simulink model "ErskineMultiDroneFormation"  (R2020b)
settings: Solver=FixedStepAuto  StartTime=0.0  StopTime=Tsim  FixedStep=sim_dt  RelTol=1e-3
values from neighbouring files (symbols this model uses):
  controller_rate = 50    [MultiQuadInit.m]
  drone_params = setDefaultDroneParams(nDrones)    [MultiQuadInit.m]
  dt_p = 0.2    [MultiQuadInit.m]    (also in setSimConditions.m)
  edges = [1,2 ... (first row only)    [MultiQuadInit.m]    (also in setSimConditions.m)
  g = 9.81    [MultiQuadInit.m]
  N_p = 5    [MultiQuadInit.m]    (also in setSimConditions.m)
  nDrones = 3    [MultiQuadInit.m]
  omega0 = zeros(3,nDrones)    [MultiQuadInit.m]    (also in setSimConditions.m)
  p0 = scale*(rand(3,nDrones) - [0.5;0.5;0])    [MultiQuadInit.m]    (also in setSimConditions.m = scale*(rand(3,nDrones) - [1/2;1/2;0]))
  q0 = zeros(4,nDrones); q0(1,:) = ones(1,nDrones)    [MultiQuadInit.m]    (also in setSimConditions.m)
  sim_dt = 0.005    [MultiQuadInit.m]
  v0 = zeros(3, nDrones)    [MultiQuadInit.m]    (also in setSimConditions.m)
undefined symbols (not defined in the file or in its folder): camera_noise
libraries: vrlib x13
(part 4 of 4)

== matlab function ErskineMultiDroneFormation/  Quadrotor13/Quadrotor/ESC ==
  data: Omega_prop_d input; prop_acceleration output; Omega_prop input; DroneID parameter; drone_params parameter
function prop_acceleration  =  ESC_ctrl(Omega_prop_d, Omega_prop, DroneID, drone_params)

prop_acceleration = (Omega_prop_d - Omega_prop)*drone_params(DroneID).motors.gain;

== matlab function ErskineMultiDroneFormation/  Quadrotor13/Quadrotor/Translation/MATLAB Function ==
  data: f input; a output; R input; g parameter; drone_params parameter; DroneID parameter
function a = fcn(f, R, g, drone_params, DroneID)
m = drone_params(DroneID).mechanical.m;
a = R*[0;0;f]/m - [0;0;g];

== matlab function ErskineMultiDroneFormation/  Quadrotor2/Controller/Controller ==
  data: u input; p input size=3; v input size=3; q input size=4; omega input size=3; thrust output size=1; moments output size=3; control_type_param parameter; drone_params parameter; DroneID parameter; g parameter
function [thrust, moments] = controller(u, p, v, q, omega, control_type_param, drone_params, DroneID, g)

  thrust = 1; % set output dim
  moments = [0;0;0]; % set output dim
  
  coder.extrinsic('droneControl'); % link simulink to matlab function
  
  % do control
  [thrust, moments] = droneControl(u, p, v, q, omega, ...
    control_type_param, drone_params, DroneID, g);

end

== matlab function ErskineMultiDroneFormation/  Quadrotor13/Quadrotor/Translation/MATLAB Function1 ==
  data: q input; R output
function R = quat2rotm(q)
  R = eye(3);
  coder.extrinsic('quat2rotm.m');
  R = quat2rotm(q);
end

== matlab function ErskineMultiDroneFormation/  Quadrotor13/Quadrotor/calculate_wrench ==
  data: Omega_props input; thrust output; moments output; drone_params parameter; DroneID parameter
function [thrust, moments] =  invAllocation(Omega_props, drone_params, DroneID)

wrench = drone_params(DroneID).control.allocation_matrix*Omega_props.^2;

thrust = wrench(1);
moments = wrench(2:4);

== matlab function ErskineMultiDroneFormation/  Quadrotor13/add_noise ==
  settings: updateMethod=DISCRETE
  data: omega input; omega_n output size=3; q input; v input; p input; q_n output size=4; v_n output size=3; p_n output size=3; drone_params parameter; DroneID parameter
function [omega_n, q_n, v_n, p_n]= add_noise(omega,q,v,p, drone_params, DroneID)

omega_n = omega + drone_params(DroneID).sensor.gyroscope_noise*(rand(3,1)-0.5);

q_n = q + drone_params(DroneID).sensor.attitude_noise*(rand(4,1)-0.5);
q_n = q_n/norm(q_n);

v_n = v + drone_params(DroneID).sensor.velocity_noise*(rand(3,1)-0.5);

p_n = p + drone_params(DroneID).sensor.position_noise*(rand(3,1)-0.5);

end

== matlab function ErskineMultiDroneFormation/  Quadrotor2/Controller/desired_prop_speed ==
  data: thrust input; Omega_props output; moment input; drone_params parameter; DroneID parameter
function Omega_props  =  Allocation(thrust, moment, drone_params, DroneID)

%  Omega_props = sqrt(inv(alloc_mat) * [thrust;moment]);
 Omega_props = real(sqrt(complex(inv(drone_params(DroneID).control.allocation_matrix) * [thrust;moment])));

== matlab function ErskineMultiDroneFormation/  Quadrotor2/Quadrotor/Attitude/MATLAB Function ==
  data: q input size=4; omega input size=3; qd output size=4
function qd  = quaternion_derivative(q, omega)


qd =  0.5 * multiplyQuaternions([0;omega],q);

end


function q = multiplyQuaternions(qA,qB)
q0 = qA(1);
q1 = qA(2);
q2 = qA(3);
q3 = qA(4);
Q = [q0, -q1, -q2, -q3;
     q1,  q0, -q3,  q2;
     q2,  q3,  q0, -q1;
     q3, -q2,  q1,  q0];
q = Q * qB;
end

== matlab function ErskineMultiDroneFormation/  Quadrotor2/Quadrotor/Attitude/MATLAB Function1 ==
  data: m input; a output; omega input; drone_params parameter; DroneID parameter
function a = moments2angularacceleration(m, omega, drone_params, DroneID)

I = drone_params(DroneID).mechanical.I;
a = inv(I)*m  - inv(I) * cross(omega,I*omega);

== matlab function ErskineMultiDroneFormation/  Quadrotor2/Quadrotor/ESC ==
  data: Omega_prop_d input; prop_acceleration output; Omega_prop input; DroneID parameter; drone_params parameter
function prop_acceleration  =  ESC_ctrl(Omega_prop_d, Omega_prop, DroneID, drone_params)

prop_acceleration = (Omega_prop_d - Omega_prop)*drone_params(DroneID).motors.gain;

== matlab function ErskineMultiDroneFormation/  Quadrotor2/Quadrotor/Translation/MATLAB Function ==
  data: f input; a output; R input; g parameter; drone_params parameter; DroneID parameter
function a = fcn(f, R, g, drone_params, DroneID)
m = drone_params(DroneID).mechanical.m;
a = R*[0;0;f]/m - [0;0;g];

== matlab function ErskineMultiDroneFormation/Formation Controller/Camera ==
  settings: updateMethod=DISCRETE
  data: States input Bus: FormationStateBus; t input; bearings output; edges parameter; noisy_bearings output; depth output; noisy_depth output; camera_noise parameter; rng_seed parameter
function [bearings, noisy_bearings,depth, noisy_depth] = Cameras(States,t, edges, camera_noise, rng_seed)
%% Cameras(States, nDrones, edges)
% [bearings, noisy_bearings,depth, noisy_depth] = Cameras(States, nDrones, edges)

%% Setup Data Structures
drones = struct2cell(States);
bearings = zeros(3, length(edges));
noisy_bearings = zeros(3, length(edges));
depth = zeros(1, length(edges));
noisy_depth = zeros(1, length(edges));

rng(rng_seed + 1000*t);

%% Calculate Bearings
for i = 1:length(edges)
  out = edges(i,1);
  in = edges(i,2);
  
  %  drone_i = drones{out};
  %  drone_j = drones{in};
  
  Ri = quat2rotm(drones{out}.q');
  dp = drones{in}.p - drones{out}.p;
  depth(i) = norm(dp);
  bearings(:,i) = Ri' * dp/depth(i);
  
  % add noise
  perp1 = cross(bearings(:,i),rand(3,1));
  perp1 = perp1/norm(perp1);
  perp2 = cross(bearings(:,i),perp1);
  perp2 = perp2/norm(perp2);
  n1 = camera_noise.perp*2*(rand(1)-0.5)*perp1;
  n2 = camera_noise.perp*2*(rand(1)-0.5)*perp2;
  noisy_bearings(:,i) = bearings(:,i) + n1 + n2;
  noisy_bearings(:,i) = noisy_bearings(:,i)/norm(noisy_bearings(:,i));
  
  noisy_depth(i) = depth(i) + camera_noise.long_bias + ...
    2*camera_noise.long*(rand(1) - 0.5);
end

end

== matlab function ErskineMultiDroneFormation/  Quadrotor3/Controller/desired_prop_speed ==
  data: thrust input; Omega_props output; moment input; drone_params parameter; DroneID parameter
function Omega_props  =  Allocation(thrust, moment, drone_params, DroneID)

%  Omega_props = sqrt(inv(alloc_mat) * [thrust;moment]);
 Omega_props = real(sqrt(complex(inv(drone_params(DroneID).control.allocation_matrix) * [thrust;moment])));

== matlab function ErskineMultiDroneFormation/  Quadrotor3/Quadrotor/Attitude/MATLAB Function ==
  data: q input size=4; omega input size=3; qd output size=4
function qd  = quaternion_derivative(q, omega)


qd =  0.5 * multiplyQuaternions([0;omega],q);

end


function q = multiplyQuaternions(qA,qB)
q0 = qA(1);
q1 = qA(2);
q2 = qA(3);
q3 = qA(4);
Q = [q0, -q1, -q2, -q3;
     q1,  q0, -q3,  q2;
     q2,  q3,  q0, -q1;
     q3, -q2,  q1,  q0];
q = Q * qB;
end

== matlab function ErskineMultiDroneFormation/  Quadrotor3/Quadrotor/Attitude/MATLAB Function1 ==
  data: m input; a output; omega input; drone_params parameter; DroneID parameter
function a = moments2angularacceleration(m, omega, drone_params, DroneID)

I = drone_params(DroneID).mechanical.I;
a = inv(I)*m  - inv(I) * cross(omega,I*omega);

== matlab function ErskineMultiDroneFormation/  Quadrotor3/Quadrotor/ESC ==
  data: Omega_prop_d input; prop_acceleration output; Omega_prop input; DroneID parameter; drone_params parameter
function prop_acceleration  =  ESC_ctrl(Omega_prop_d, Omega_prop, DroneID, drone_params)

prop_acceleration = (Omega_prop_d - Omega_prop)*drone_params(DroneID).motors.gain;

== matlab function ErskineMultiDroneFormation/  Quadrotor1/Controller/Controller ==
  data: u input; p input size=3; v input size=3; q input size=4; omega input size=3; thrust output size=1; moments output size=3; control_type_param parameter; drone_params parameter; DroneID parameter; g parameter
function [thrust, moments] = controller(u, p, v, q, omega, control_type_param, drone_params, DroneID, g)

  thrust = 1; % set output dim
  moments = [0;0;0]; % set output dim
  
  coder.extrinsic('droneControl'); % link simulink to matlab function
  
  % do control
  [thrust, moments] = droneControl(u, p, v, q, omega, ...
    control_type_param, drone_params, DroneID, g);

end

== matlab function ErskineMultiDroneFormation/  Quadrotor3/Quadrotor/Translation/MATLAB Function ==
  data: f input; a output; R input; g parameter; drone_params parameter; DroneID parameter
function a = fcn(f, R, g, drone_params, DroneID)
m = drone_params(DroneID).mechanical.m;
a = R*[0;0;f]/m - [0;0;g];

== matlab function ErskineMultiDroneFormation/  Quadrotor3/Quadrotor/Translation/MATLAB Function1 ==
  data: q input; R output
function R = quat2rotm(q)
  R = eye(3);
  coder.extrinsic('quat2rotm.m');
  R = quat2rotm(q);
end

== matlab function ErskineMultiDroneFormation/  Quadrotor3/Quadrotor/calculate_wrench ==
  data: Omega_props input; thrust output; moments output; drone_params parameter; DroneID parameter
function [thrust, moments] =  invAllocation(Omega_props, drone_params, DroneID)

wrench = drone_params(DroneID).control.allocation_matrix*Omega_props.^2;

thrust = wrench(1);
moments = wrench(2:4);

== matlab function ErskineMultiDroneFormation/  Quadrotor3/add_noise ==
  settings: updateMethod=DISCRETE
  data: omega input; omega_n output size=3; q input; v input; p input; q_n output size=4; v_n output size=3; p_n output size=3; drone_params parameter; DroneID parameter
function [omega_n, q_n, v_n, p_n]= add_noise(omega,q,v,p, drone_params, DroneID)

omega_n = omega + drone_params(DroneID).sensor.gyroscope_noise*(rand(3,1)-0.5);

q_n = q + drone_params(DroneID).sensor.attitude_noise*(rand(4,1)-0.5);
q_n = q_n/norm(q_n);

v_n = v + drone_params(DroneID).sensor.velocity_noise*(rand(3,1)-0.5);

p_n = p + drone_params(DroneID).sensor.position_noise*(rand(3,1)-0.5);

end

== matlab function ErskineMultiDroneFormation/Formation Controller/FormationControlFunction ==
  data: states input Bus: FormationStateBus; out output size=[4*nDrones]; B_desired input; B_forward input; B_measure input; d_measure input; init_guess input; nDrones parameter; result output; N_p parameter; dt_p parameter; edges parameter; control_type parameter
function [out, result] = FormationControlFunction(states, B_desired, B_forward, B_measure, d_measure, init_guess, nDrones, N_p, dt_p, edges, control_type)
%% ControlFunction
% the control u of a drone consists of [fz; omega]
% the output of this block is  out = [u1; u2; un]
% the result of a drone is [fz1; omega1; ...; fzn, omegan]
% the result of thisblock is [result1; ...; resultn]

% Determine if first iteration
if max(init_guess) < 0.001
  first_iter = true;
else
  first_iter = false;
end


% Function variables setup
out = zeros(nDrones*4,1);
result = init_guess;

coder.extrinsic('GradientBearingController');
coder.extrinsic('ForwardMPCFormationControl');
coder.extrinsic('CommunicatingMPCFormationControl');


%% Do Control
if control_type == 1 % Gradient Controller
  if first_iter
    disp(['Control type: Gradient'])
  end
  out = GradientBearingController(B_measure, B_desired, states, nDrones, edges);
  result = ones(nDrones*4*N_p, 1);
elseif control_type == 2 % Forward Desired MPC
  if first_iter
    for i = 1:4:length(init_guess)
      init_guess(i) = 10;
    end
    disp(['Control type: Forward MPC'])
  end
  [out, result] = ForwardMPCFormationControl(states, B_forward, B_measure, d_measure, init_guess, nDrones, N_p, dt_p, edges);
elseif control_type == 3 % Forward Desired MPC with Communication
  if first_iter
    for i = 1:4:length(init_guess)
      init_guess(i) = 10;
    end
    disp(['Control type: Forward MPC with Full Communication'])
  end
  [out, result] = CommunicatingMPCFormationControl(states, B_forward, B_measure, d_measure, init_guess, nDrones, N_p, dt_p, edges);
else
  error("Chosen Control Type is Invalid")
end


%% Processing of Results

return

== matlab function ErskineMultiDroneFormation/  Quadrotor2/Quadrotor/Translation/MATLAB Function1 ==
  data: q input; R output
function R = quat2rotm(q)
  R = eye(3);
  coder.extrinsic('quat2rotm.m');
  R = quat2rotm(q);
end

== matlab function ErskineMultiDroneFormation/  Quadrotor2/Quadrotor/calculate_wrench ==
  data: Omega_props input; thrust output; moments output; drone_params parameter; DroneID parameter
function [thrust, moments] =  invAllocation(Omega_props, drone_params, DroneID)

wrench = drone_params(DroneID).control.allocation_matrix*Omega_props.^2;

thrust = wrench(1);
moments = wrench(2:4);

== matlab function ErskineMultiDroneFormation/  Quadrotor2/add_noise ==
  settings: updateMethod=DISCRETE
  data: omega input; omega_n output size=3; q input; v input; p input; q_n output size=4; v_n output size=3; p_n output size=3; drone_params parameter; DroneID parameter
function [omega_n, q_n, v_n, p_n]= add_noise(omega,q,v,p, drone_params, DroneID)

omega_n = omega + drone_params(DroneID).sensor.gyroscope_noise*(rand(3,1)-0.5);

q_n = q + drone_params(DroneID).sensor.attitude_noise*(rand(4,1)-0.5);
q_n = q_n/norm(q_n);

v_n = v + drone_params(DroneID).sensor.velocity_noise*(rand(3,1)-0.5);

p_n = p + drone_params(DroneID).sensor.position_noise*(rand(3,1)-0.5);

end

== matlab function ErskineMultiDroneFormation/  Quadrotor4/Controller/Controller ==
  data: u input; p input size=3; v input size=3; q input size=4; omega input size=3; thrust output size=1; moments output size=3; control_type_param parameter; drone_params parameter; DroneID parameter; g parameter
function [thrust, moments] = controller(u, p, v, q, omega, control_type_param, drone_params, DroneID, g)

  thrust = 1; % set output dim
  moments = [0;0;0]; % set output dim
  
  coder.extrinsic('droneControl'); % link simulink to matlab function
  
  % do control
  [thrust, moments] = droneControl(u, p, v, q, omega, ...
    control_type_param, drone_params, DroneID, g);

end

== matlab function ErskineMultiDroneFormation/  Quadrotor4/Controller/desired_prop_speed ==
  data: thrust input; Omega_props output; moment input; drone_params parameter; DroneID parameter
function Omega_props  =  Allocation(thrust, moment, drone_params, DroneID)

%  Omega_props = sqrt(inv(alloc_mat) * [thrust;moment]);
 Omega_props = real(sqrt(complex(inv(drone_params(DroneID).control.allocation_matrix) * [thrust;moment])));

== matlab function ErskineMultiDroneFormation/  Quadrotor4/Quadrotor/Attitude/MATLAB Function ==
  data: q input size=4; omega input size=3; qd output size=4
function qd  = quaternion_derivative(q, omega)


qd =  0.5 * multiplyQuaternions([0;omega],q);

end


function q = multiplyQuaternions(qA,qB)
q0 = qA(1);
q1 = qA(2);
q2 = qA(3);
q3 = qA(4);
Q = [q0, -q1, -q2, -q3;
     q1,  q0, -q3,  q2;
     q2,  q3,  q0, -q1;
     q3, -q2,  q1,  q0];
q = Q * qB;
end

== matlab function ErskineMultiDroneFormation/  Quadrotor4/Quadrotor/Attitude/MATLAB Function1 ==
  data: m input; a output; omega input; drone_params parameter; DroneID parameter
function a = moments2angularacceleration(m, omega, drone_params, DroneID)

I = drone_params(DroneID).mechanical.I;
a = inv(I)*m  - inv(I) * cross(omega,I*omega);

== matlab function ErskineMultiDroneFormation/  Quadrotor4/Quadrotor/ESC ==
  data: Omega_prop_d input; prop_acceleration output; Omega_prop input; DroneID parameter; drone_params parameter
function prop_acceleration  =  ESC_ctrl(Omega_prop_d, Omega_prop, DroneID, drone_params)

prop_acceleration = (Omega_prop_d - Omega_prop)*drone_params(DroneID).motors.gain;

== matlab function ErskineMultiDroneFormation/  Quadrotor4/Quadrotor/Translation/MATLAB Function ==
  data: f input; a output; R input; g parameter; drone_params parameter; DroneID parameter
function a = fcn(f, R, g, drone_params, DroneID)
m = drone_params(DroneID).mechanical.m;
a = R*[0;0;f]/m - [0;0;g];

== matlab function ErskineMultiDroneFormation/  Quadrotor1/Controller/desired_prop_speed ==
  data: thrust input; Omega_props output; moment input; drone_params parameter; DroneID parameter
function Omega_props  =  Allocation(thrust, moment, drone_params, DroneID)

%  Omega_props = sqrt(inv(alloc_mat) * [thrust;moment]);
 Omega_props = real(sqrt(complex(inv(drone_params(DroneID).control.allocation_matrix) * [thrust;moment])));

== matlab function ErskineMultiDroneFormation/  Quadrotor4/Quadrotor/Translation/MATLAB Function1 ==
  data: q input; R output
function R = quat2rotm(q)
  R = eye(3);
  coder.extrinsic('quat2rotm.m');
  R = quat2rotm(q);
end

== matlab function ErskineMultiDroneFormation/  Quadrotor4/Quadrotor/calculate_wrench ==
  data: Omega_props input; thrust output; moments output; drone_params parameter; DroneID parameter
function [thrust, moments] =  invAllocation(Omega_props, drone_params, DroneID)

wrench = drone_params(DroneID).control.allocation_matrix*Omega_props.^2;

thrust = wrench(1);
moments = wrench(2:4);

== matlab function ErskineMultiDroneFormation/  Quadrotor4/add_noise ==
  settings: updateMethod=DISCRETE
  data: omega input; omega_n output size=3; q input; v input; p input; q_n output size=4; v_n output size=3; p_n output size=3; drone_params parameter; DroneID parameter
function [omega_n, q_n, v_n, p_n]= add_noise(omega,q,v,p, drone_params, DroneID)

omega_n = omega + drone_params(DroneID).sensor.gyroscope_noise*(rand(3,1)-0.5);

q_n = q + drone_params(DroneID).sensor.attitude_noise*(rand(4,1)-0.5);
q_n = q_n/norm(q_n);

v_n = v + drone_params(DroneID).sensor.velocity_noise*(rand(3,1)-0.5);

p_n = p + drone_params(DroneID).sensor.position_noise*(rand(3,1)-0.5);

end

== matlab function ErskineMultiDroneFormation/  Quadrotor5/Controller/Controller ==
  data: u input; p input size=3; v input size=3; q input size=4; omega input size=3; thrust output size=1; moments output size=3; control_type_param parameter; drone_params parameter; DroneID parameter; g parameter
function [thrust, moments] = controller(u, p, v, q, omega, control_type_param, drone_params, DroneID, g)

  thrust = 1; % set output dim
  moments = [0;0;0]; % set output dim
  
  coder.extrinsic('droneControl'); % link simulink to matlab function
  
  % do control
  [thrust, moments] = droneControl(u, p, v, q, omega, ...
    control_type_param, drone_params, DroneID, g);

end

== matlab function ErskineMultiDroneFormation/  Quadrotor5/Controller/desired_prop_speed ==
  data: thrust input; Omega_props output; moment input; drone_params parameter; DroneID parameter
function Omega_props  =  Allocation(thrust, moment, drone_params, DroneID)

%  Omega_props = sqrt(inv(alloc_mat) * [thrust;moment]);
 Omega_props = real(sqrt(complex(inv(drone_params(DroneID).control.allocation_matrix) * [thrust;moment])));

== matlab function ErskineMultiDroneFormation/  Quadrotor5/Quadrotor/Attitude/MATLAB Function ==
  data: q input size=4; omega input size=3; qd output size=4
function qd  = quaternion_derivative(q, omega)


qd =  0.5 * multiplyQuaternions([0;omega],q);

end


function q = multiplyQuaternions(qA,qB)
q0 = qA(1);
q1 = qA(2);
q2 = qA(3);
q3 = qA(4);
Q = [q0, -q1, -q2, -q3;
     q1,  q0, -q3,  q2;
     q2,  q3,  q0, -q1;
     q3, -q2,  q1,  q0];
q = Q * qB;
end

== matlab function ErskineMultiDroneFormation/  Quadrotor5/Quadrotor/Attitude/MATLAB Function1 ==
  data: m input; a output; omega input; drone_params parameter; DroneID parameter
function a = moments2angularacceleration(m, omega, drone_params, DroneID)

I = drone_params(DroneID).mechanical.I;
a = inv(I)*m  - inv(I) * cross(omega,I*omega);

== matlab function ErskineMultiDroneFormation/  Quadrotor5/Quadrotor/ESC ==
  data: Omega_prop_d input; prop_acceleration output; Omega_prop input; DroneID parameter; drone_params parameter
function prop_acceleration  =  ESC_ctrl(Omega_prop_d, Omega_prop, DroneID, drone_params)

prop_acceleration = (Omega_prop_d - Omega_prop)*drone_params(DroneID).motors.gain;

== matlab function ErskineMultiDroneFormation/  Quadrotor5/Quadrotor/Translation/MATLAB Function ==
  data: f input; a output; R input; g parameter; drone_params parameter; DroneID parameter
function a = fcn(f, R, g, drone_params, DroneID)
m = drone_params(DroneID).mechanical.m;
a = R*[0;0;f]/m - [0;0;g];

== matlab function ErskineMultiDroneFormation/  Quadrotor1/Quadrotor/Attitude/MATLAB Function ==
  data: q input size=4; omega input size=3; qd output size=4
function qd  = quaternion_derivative(q, omega)


qd =  0.5 * multiplyQuaternions([0;omega],q);

end


function q = multiplyQuaternions(qA,qB)
q0 = qA(1);
q1 = qA(2);
q2 = qA(3);
q3 = qA(4);
Q = [q0, -q1, -q2, -q3;
     q1,  q0, -q3,  q2;
     q2,  q3,  q0, -q1;
     q3, -q2,  q1,  q0];
q = Q * qB;
end

== matlab function ErskineMultiDroneFormation/  Quadrotor5/Quadrotor/Translation/MATLAB Function1 ==
  data: q input; R output
function R = quat2rotm(q)
  R = eye(3);
  coder.extrinsic('quat2rotm.m');
  R = quat2rotm(q);
end

== matlab function ErskineMultiDroneFormation/  Quadrotor5/Quadrotor/calculate_wrench ==
  data: Omega_props input; thrust output; moments output; drone_params parameter; DroneID parameter
function [thrust, moments] =  invAllocation(Omega_props, drone_params, DroneID)

wrench = drone_params(DroneID).control.allocation_matrix*Omega_props.^2;

thrust = wrench(1);
moments = wrench(2:4);

== matlab function ErskineMultiDroneFormation/  Quadrotor5/add_noise ==
  settings: updateMethod=DISCRETE
  data: omega input; omega_n output size=3; q input; v input; p input; q_n output size=4; v_n output size=3; p_n output size=3; drone_params parameter; DroneID parameter
function [omega_n, q_n, v_n, p_n]= add_noise(omega,q,v,p, drone_params, DroneID)

omega_n = omega + drone_params(DroneID).sensor.gyroscope_noise*(rand(3,1)-0.5);

q_n = q + drone_params(DroneID).sensor.attitude_noise*(rand(4,1)-0.5);
q_n = q_n/norm(q_n);

v_n = v + drone_params(DroneID).sensor.velocity_noise*(rand(3,1)-0.5);

p_n = p + drone_params(DroneID).sensor.position_noise*(rand(3,1)-0.5);

end

== matlab function ErskineMultiDroneFormation/  Quadrotor6/Controller/Controller ==
  data: u input; p input size=3; v input size=3; q input size=4; omega input size=3; thrust output size=1; moments output size=3; control_type_param parameter; drone_params parameter; DroneID parameter; g parameter
function [thrust, moments] = controller(u, p, v, q, omega, control_type_param, drone_params, DroneID, g)

  thrust = 1; % set output dim
  moments = [0;0;0]; % set output dim
  
  coder.extrinsic('droneControl'); % link simulink to matlab function
  
  % do control
  [thrust, moments] = droneControl(u, p, v, q, omega, ...
    control_type_param, drone_params, DroneID, g);

end

== matlab function ErskineMultiDroneFormation/  Quadrotor6/Controller/desired_prop_speed ==
  data: thrust input; Omega_props output; moment input; drone_params parameter; DroneID parameter
function Omega_props  =  Allocation(thrust, moment, drone_params, DroneID)

%  Omega_props = sqrt(inv(alloc_mat) * [thrust;moment]);
 Omega_props = real(sqrt(complex(inv(drone_params(DroneID).control.allocation_matrix) * [thrust;moment])));

== matlab function ErskineMultiDroneFormation/  Quadrotor6/Quadrotor/Attitude/MATLAB Function ==
  data: q input size=4; omega input size=3; qd output size=4
function qd  = quaternion_derivative(q, omega)


qd =  0.5 * multiplyQuaternions([0;omega],q);

end


function q = multiplyQuaternions(qA,qB)
q0 = qA(1);
q1 = qA(2);
q2 = qA(3);
q3 = qA(4);
Q = [q0, -q1, -q2, -q3;
     q1,  q0, -q3,  q2;
     q2,  q3,  q0, -q1;
     q3, -q2,  q1,  q0];
q = Q * qB;
end

== matlab function ErskineMultiDroneFormation/  Quadrotor6/Quadrotor/Attitude/MATLAB Function1 ==
  data: m input; a output; omega input; drone_params parameter; DroneID parameter
function a = moments2angularacceleration(m, omega, drone_params, DroneID)

I = drone_params(DroneID).mechanical.I;
a = inv(I)*m  - inv(I) * cross(omega,I*omega);

== matlab function ErskineMultiDroneFormation/  Quadrotor6/Quadrotor/ESC ==
  data: Omega_prop_d input; prop_acceleration output; Omega_prop input; DroneID parameter; drone_params parameter
function prop_acceleration  =  ESC_ctrl(Omega_prop_d, Omega_prop, DroneID, drone_params)

prop_acceleration = (Omega_prop_d - Omega_prop)*drone_params(DroneID).motors.gain;

== matlab function ErskineMultiDroneFormation/  Quadrotor1/Quadrotor/Attitude/MATLAB Function1 ==
  data: m input; a output; omega input; drone_params parameter; DroneID parameter
function a = moments2angularacceleration(m, omega, drone_params, DroneID)

I = drone_params(DroneID).mechanical.I;
a = inv(I)*m  - inv(I) * cross(omega,I*omega);

== matlab function ErskineMultiDroneFormation/  Quadrotor6/Quadrotor/Translation/MATLAB Function ==
  data: f input; a output; R input; g parameter; drone_params parameter; DroneID parameter
function a = fcn(f, R, g, drone_params, DroneID)
m = drone_params(DroneID).mechanical.m;
a = R*[0;0;f]/m - [0;0;g];

== matlab function ErskineMultiDroneFormation/  Quadrotor6/Quadrotor/Translation/MATLAB Function1 ==
  data: q input; R output
function R = quat2rotm(q)
  R = eye(3);
  coder.extrinsic('quat2rotm.m');
  R = quat2rotm(q);
end

== matlab function ErskineMultiDroneFormation/  Quadrotor6/Quadrotor/calculate_wrench ==
  data: Omega_props input; thrust output; moments output; drone_params parameter; DroneID parameter
function [thrust, moments] =  invAllocation(Omega_props, drone_params, DroneID)

wrench = drone_params(DroneID).control.allocation_matrix*Omega_props.^2;

thrust = wrench(1);
moments = wrench(2:4);

== matlab function ErskineMultiDroneFormation/  Quadrotor6/add_noise ==
  settings: updateMethod=DISCRETE
  data: omega input; omega_n output size=3; q input; v input; p input; q_n output size=4; v_n output size=3; p_n output size=3; drone_params parameter; DroneID parameter
function [omega_n, q_n, v_n, p_n]= add_noise(omega,q,v,p, drone_params, DroneID)

omega_n = omega + drone_params(DroneID).sensor.gyroscope_noise*(rand(3,1)-0.5);

q_n = q + drone_params(DroneID).sensor.attitude_noise*(rand(4,1)-0.5);
q_n = q_n/norm(q_n);

v_n = v + drone_params(DroneID).sensor.velocity_noise*(rand(3,1)-0.5);

p_n = p + drone_params(DroneID).sensor.position_noise*(rand(3,1)-0.5);

end

== matlab function ErskineMultiDroneFormation/Formation Controller1/Camera ==
  settings: updateMethod=DISCRETE
  data: States input Bus: FormationStateBus; t input; bearings output; edges parameter; noisy_bearings output; depth output; noisy_depth output; camera_noise parameter; rng_seed parameter
function [bearings, noisy_bearings,depth, noisy_depth] = Cameras(States,t, edges, camera_noise, rng_seed)
%% Cameras(States, nDrones, edges)
% [bearings, noisy_bearings,depth, noisy_depth] = Cameras(States, nDrones, edges)

%% Setup Data Structures
drones = struct2cell(States);
bearings = zeros(3, length(edges));
noisy_bearings = zeros(3, length(edges));
depth = zeros(1, length(edges));
noisy_depth = zeros(1, length(edges));

rng(rng_seed + 1000*t);

%% Calculate Bearings
for i = 1:length(edges)
  out = edges(i,1);
  in = edges(i,2);
  
  %  drone_i = drones{out};
  %  drone_j = drones{in};
  
  Ri = quat2rotm(drones{out}.q');
  dp = drones{in}.p - drones{out}.p;
  depth(i) = norm(dp);
  bearings(:,i) = Ri' * dp/depth(i);
  
  % add noise
  perp1 = cross(bearings(:,i),rand(3,1));
  perp1 = perp1/norm(perp1);
  perp2 = cross(bearings(:,i),perp1);
  perp2 = perp2/norm(perp2);
  n1 = camera_noise.perp*2*(rand(1)-0.5)*perp1;
  n2 = camera_noise.perp*2*(rand(1)-0.5)*perp2;
  noisy_bearings(:,i) = bearings(:,i) + n1 + n2;
  noisy_bearings(:,i) = noisy_bearings(:,i)/norm(noisy_bearings(:,i));
  
  noisy_depth(i) = depth(i) + camera_noise.long_bias + ...
    2*camera_noise.long*(rand(1) - 0.5);
end

end

== matlab function ErskineMultiDroneFormation/Formation Controller1/FormationControlFunction ==
  data: states input Bus: FormationStateBus; out output size=[4*nDrones]; B_desired input; B_forward input; B_measure input; d_measure input; init_guess input; nDrones parameter; result output; N_p parameter; dt_p parameter; edges parameter; control_type parameter
function [out, result] = FormationControlFunction(states, B_desired, B_forward, B_measure, d_measure, init_guess, nDrones, N_p, dt_p, edges, control_type)
%% ControlFunction
% the control u of a drone consists of [fz; omega]
% the output of this block is  out = [u1; u2; un]
% the result of a drone is [fz1; omega1; ...; fzn, omegan]
% the result of thisblock is [result1; ...; resultn]

% Determine if first iteration
if max(init_guess) < 0.001
  first_iter = true;
else
  first_iter = false;
end


% Function variables setup
out = zeros(nDrones*4,1);
result = init_guess;

coder.extrinsic('GradientBearingController');
coder.extrinsic('ForwardMPCFormationControl');
coder.extrinsic('CommunicatingMPCFormationControl');


%% Do Control
if control_type == 1 % Gradient Controller
  if first_iter
    disp(['Control type: Gradient'])
  end
  out = GradientBearingController(B_measure, B_desired, states, nDrones, edges);
  result = ones(nDrones*4*N_p, 1);
elseif control_type == 2 % Forward Desired MPC
  if first_iter
    for i = 1:4:length(init_guess)
      init_guess(i) = 10;
    end
    disp(['Control type: Forward MPC'])
  end
  [out, result] = ForwardMPCFormationControl(states, B_forward, B_measure, d_measure, init_guess, nDrones, N_p, dt_p, edges);
elseif control_type == 3 % Forward Desired MPC with Communication
  if first_iter
    for i = 1:4:length(init_guess)
      init_guess(i) = 10;
    end
    disp(['Control type: Forward MPC with Full Communication'])
  end
  [out, result] = CommunicatingMPCFormationControl(states, B_forward, B_measure, d_measure, init_guess, nDrones, N_p, dt_p, edges);
else
  error("Chosen Control Type is Invalid")
end


%% Processing of Results

return

== matlab function ErskineMultiDroneFormation/  Quadrotor7/Controller/Controller ==
  data: u input; p input size=3; v input size=3; q input size=4; omega input size=3; thrust output size=1; moments output size=3; control_type_param parameter; drone_params parameter; DroneID parameter; g parameter
function [thrust, moments] = controller(u, p, v, q, omega, control_type_param, drone_params, DroneID, g)

  thrust = 1; % set output dim
  moments = [0;0;0]; % set output dim
  
  coder.extrinsic('droneControl'); % link simulink to matlab function
  
  % do control
  [thrust, moments] = droneControl(u, p, v, q, omega, ...
    control_type_param, drone_params, DroneID, g);

end

== matlab function ErskineMultiDroneFormation/  Quadrotor7/Controller/desired_prop_speed ==
  data: thrust input; Omega_props output; moment input; drone_params parameter; DroneID parameter
function Omega_props  =  Allocation(thrust, moment, drone_params, DroneID)

%  Omega_props = sqrt(inv(alloc_mat) * [thrust;moment]);
 Omega_props = real(sqrt(complex(inv(drone_params(DroneID).control.allocation_matrix) * [thrust;moment])));

== matlab function ErskineMultiDroneFormation/  Quadrotor1/Quadrotor/ESC ==
  data: Omega_prop_d input; prop_acceleration output; Omega_prop input; DroneID parameter; drone_params parameter
function prop_acceleration  =  ESC_ctrl(Omega_prop_d, Omega_prop, DroneID, drone_params)

prop_acceleration = (Omega_prop_d - Omega_prop)*drone_params(DroneID).motors.gain;

== matlab function ErskineMultiDroneFormation/  Quadrotor7/Quadrotor/Attitude/MATLAB Function ==
  data: q input size=4; omega input size=3; qd output size=4
function qd  = quaternion_derivative(q, omega)


qd =  0.5 * multiplyQuaternions([0;omega],q);

end


function q = multiplyQuaternions(qA,qB)
q0 = qA(1);
q1 = qA(2);
q2 = qA(3);
q3 = qA(4);
Q = [q0, -q1, -q2, -q3;
     q1,  q0, -q3,  q2;
     q2,  q3,  q0, -q1;
     q3, -q2,  q1,  q0];
q = Q * qB;
end

== matlab function ErskineMultiDroneFormation/  Quadrotor7/Quadrotor/Attitude/MATLAB Function1 ==
  data: m input; a output; omega input; drone_params parameter; DroneID parameter
function a = moments2angularacceleration(m, omega, drone_params, DroneID)

I = drone_params(DroneID).mechanical.I;
a = inv(I)*m  - inv(I) * cross(omega,I*omega);

== matlab function ErskineMultiDroneFormation/  Quadrotor7/Quadrotor/ESC ==
  data: Omega_prop_d input; prop_acceleration output; Omega_prop input; DroneID parameter; drone_params parameter
function prop_acceleration  =  ESC_ctrl(Omega_prop_d, Omega_prop, DroneID, drone_params)

prop_acceleration = (Omega_prop_d - Omega_prop)*drone_params(DroneID).motors.gain;

== matlab function ErskineMultiDroneFormation/  Quadrotor7/Quadrotor/Translation/MATLAB Function ==
  data: f input; a output; R input; g parameter; drone_params parameter; DroneID parameter
function a = fcn(f, R, g, drone_params, DroneID)
m = drone_params(DroneID).mechanical.m;
a = R*[0;0;f]/m - [0;0;g];

== matlab function ErskineMultiDroneFormation/  Quadrotor7/Quadrotor/Translation/MATLAB Function1 ==
  data: q input; R output
function R = quat2rotm(q)
  R = eye(3);
  coder.extrinsic('quat2rotm.m');
  R = quat2rotm(q);
end

== matlab function ErskineMultiDroneFormation/  Quadrotor7/Quadrotor/calculate_wrench ==
  data: Omega_props input; thrust output; moments output; drone_params parameter; DroneID parameter
function [thrust, moments] =  invAllocation(Omega_props, drone_params, DroneID)

wrench = drone_params(DroneID).control.allocation_matrix*Omega_props.^2;

thrust = wrench(1);
moments = wrench(2:4);

== matlab function ErskineMultiDroneFormation/  Quadrotor7/add_noise ==
  settings: updateMethod=DISCRETE
  data: omega input; omega_n output size=3; q input; v input; p input; q_n output size=4; v_n output size=3; p_n output size=3; drone_params parameter; DroneID parameter
function [omega_n, q_n, v_n, p_n]= add_noise(omega,q,v,p, drone_params, DroneID)

omega_n = omega + drone_params(DroneID).sensor.gyroscope_noise*(rand(3,1)-0.5);

q_n = q + drone_params(DroneID).sensor.attitude_noise*(rand(4,1)-0.5);
q_n = q_n/norm(q_n);

v_n = v + drone_params(DroneID).sensor.velocity_noise*(rand(3,1)-0.5);

p_n = p + drone_params(DroneID).sensor.position_noise*(rand(3,1)-0.5);

end

== matlab function ErskineMultiDroneFormation/  Quadrotor8/Controller/Controller ==
  data: u input; p input size=3; v input size=3; q input size=4; omega input size=3; thrust output size=1; moments output size=3; control_type_param parameter; drone_params parameter; DroneID parameter; g parameter
function [thrust, moments] = controller(u, p, v, q, omega, control_type_param, drone_params, DroneID, g)

  thrust = 1; % set output dim
  moments = [0;0;0]; % set output dim
  
  coder.extrinsic('droneControl'); % link simulink to matlab function
  
  % do control
  [thrust, moments] = droneControl(u, p, v, q, omega, ...
    control_type_param, drone_params, DroneID, g);

end

== matlab function ErskineMultiDroneFormation/  Quadrotor8/Controller/desired_prop_speed ==
  data: thrust input; Omega_props output; moment input; drone_params parameter; DroneID parameter
function Omega_props  =  Allocation(thrust, moment, drone_params, DroneID)

%  Omega_props = sqrt(inv(alloc_mat) * [thrust;moment]);
 Omega_props = real(sqrt(complex(inv(drone_params(DroneID).control.allocation_matrix) * [thrust;moment])));

== matlab function ErskineMultiDroneFormation/  Quadrotor1/Quadrotor/Translation/MATLAB Function ==
  data: f input; a output; R input; g parameter; drone_params parameter; DroneID parameter
function a = fcn(f, R, g, drone_params, DroneID)
m = drone_params(DroneID).mechanical.m;
a = R*[0;0;f]/m - [0;0;g];

== matlab function ErskineMultiDroneFormation/  Quadrotor8/Quadrotor/Attitude/MATLAB Function ==
  data: q input size=4; omega input size=3; qd output size=4
function qd  = quaternion_derivative(q, omega)


qd =  0.5 * multiplyQuaternions([0;omega],q);

end


function q = multiplyQuaternions(qA,qB)
q0 = qA(1);
q1 = qA(2);
q2 = qA(3);
q3 = qA(4);
Q = [q0, -q1, -q2, -q3;
     q1,  q0, -q3,  q2;
     q2,  q3,  q0, -q1;
     q3, -q2,  q1,  q0];
q = Q * qB;
end

== matlab function ErskineMultiDroneFormation/  Quadrotor8/Quadrotor/Attitude/MATLAB Function1 ==
  data: m input; a output; omega input; drone_params parameter; DroneID parameter
function a = moments2angularacceleration(m, omega, drone_params, DroneID)

I = drone_params(DroneID).mechanical.I;
a = inv(I)*m  - inv(I) * cross(omega,I*omega);

== matlab function ErskineMultiDroneFormation/  Quadrotor8/Quadrotor/ESC ==
  data: Omega_prop_d input; prop_acceleration output; Omega_prop input; DroneID parameter; drone_params parameter
function prop_acceleration  =  ESC_ctrl(Omega_prop_d, Omega_prop, DroneID, drone_params)

prop_acceleration = (Omega_prop_d - Omega_prop)*drone_params(DroneID).motors.gain;

== matlab function ErskineMultiDroneFormation/  Quadrotor8/Quadrotor/Translation/MATLAB Function ==
  data: f input; a output; R input; g parameter; drone_params parameter; DroneID parameter
function a = fcn(f, R, g, drone_params, DroneID)
m = drone_params(DroneID).mechanical.m;
a = R*[0;0;f]/m - [0;0;g];

== matlab function ErskineMultiDroneFormation/  Quadrotor8/Quadrotor/Translation/MATLAB Function1 ==
  data: q input; R output
function R = quat2rotm(q)
  R = eye(3);
  coder.extrinsic('quat2rotm.m');
  R = quat2rotm(q);
end

== matlab function ErskineMultiDroneFormation/  Quadrotor8/Quadrotor/calculate_wrench ==
  data: Omega_props input; thrust output; moments output; drone_params parameter; DroneID parameter
function [thrust, moments] =  invAllocation(Omega_props, drone_params, DroneID)

wrench = drone_params(DroneID).control.allocation_matrix*Omega_props.^2;

thrust = wrench(1);
moments = wrench(2:4);

== matlab function ErskineMultiDroneFormation/  Quadrotor8/add_noise ==
  settings: updateMethod=DISCRETE
  data: omega input; omega_n output size=3; q input; v input; p input; q_n output size=4; v_n output size=3; p_n output size=3; drone_params parameter; DroneID parameter
function [omega_n, q_n, v_n, p_n]= add_noise(omega,q,v,p, drone_params, DroneID)

omega_n = omega + drone_params(DroneID).sensor.gyroscope_noise*(rand(3,1)-0.5);

q_n = q + drone_params(DroneID).sensor.attitude_noise*(rand(4,1)-0.5);
q_n = q_n/norm(q_n);

v_n = v + drone_params(DroneID).sensor.velocity_noise*(rand(3,1)-0.5);

p_n = p + drone_params(DroneID).sensor.position_noise*(rand(3,1)-0.5);

end

== matlab function ErskineMultiDroneFormation/  Quadrotor9/Controller/Controller ==
  data: u input; p input size=3; v input size=3; q input size=4; omega input size=3; thrust output size=1; moments output size=3; control_type_param parameter; drone_params parameter; DroneID parameter; g parameter
function [thrust, moments] = controller(u, p, v, q, omega, control_type_param, drone_params, DroneID, g)

  thrust = 1; % set output dim
  moments = [0;0;0]; % set output dim
  
  coder.extrinsic('droneControl'); % link simulink to matlab function
  
  % do control
  [thrust, moments] = droneControl(u, p, v, q, omega, ...
    control_type_param, drone_params, DroneID, g);

end

== matlab function ErskineMultiDroneFormation/  Quadrotor9/Controller/desired_prop_speed ==
  data: thrust input; Omega_props output; moment input; drone_params parameter; DroneID parameter
function Omega_props  =  Allocation(thrust, moment, drone_params, DroneID)

%  Omega_props = sqrt(inv(alloc_mat) * [thrust;moment]);
 Omega_props = real(sqrt(complex(inv(drone_params(DroneID).control.allocation_matrix) * [thrust;moment])));

== matlab function ErskineMultiDroneFormation/  Quadrotor9/Quadrotor/Attitude/MATLAB Function ==
  data: q input size=4; omega input size=3; qd output size=4
function qd  = quaternion_derivative(q, omega)


qd =  0.5 * multiplyQuaternions([0;omega],q);

end


function q = multiplyQuaternions(qA,qB)
q0 = qA(1);
q1 = qA(2);
q2 = qA(3);
q3 = qA(4);
Q = [q0, -q1, -q2, -q3;
     q1,  q0, -q3,  q2;
     q2,  q3,  q0, -q1;
     q3, -q2,  q1,  q0];
q = Q * qB;
end

== matlab function ErskineMultiDroneFormation/  Quadrotor9/Quadrotor/Attitude/MATLAB Function1 ==
  data: m input; a output; omega input; drone_params parameter; DroneID parameter
function a = moments2angularacceleration(m, omega, drone_params, DroneID)

I = drone_params(DroneID).mechanical.I;
a = inv(I)*m  - inv(I) * cross(omega,I*omega);

== matlab function ErskineMultiDroneFormation/  Quadrotor1/Quadrotor/Translation/MATLAB Function1 ==
  data: q input; R output
function R = quat2rotm(q)
  R = eye(3);
  coder.extrinsic('quat2rotm.m');
  R = quat2rotm(q);
end

== matlab function ErskineMultiDroneFormation/  Quadrotor9/Quadrotor/ESC ==
  data: Omega_prop_d input; prop_acceleration output; Omega_prop input; DroneID parameter; drone_params parameter
function prop_acceleration  =  ESC_ctrl(Omega_prop_d, Omega_prop, DroneID, drone_params)

prop_acceleration = (Omega_prop_d - Omega_prop)*drone_params(DroneID).motors.gain;

== matlab function ErskineMultiDroneFormation/  Quadrotor9/Quadrotor/Translation/MATLAB Function ==
  data: f input; a output; R input; g parameter; drone_params parameter; DroneID parameter
function a = fcn(f, R, g, drone_params, DroneID)
m = drone_params(DroneID).mechanical.m;
a = R*[0;0;f]/m - [0;0;g];

== matlab function ErskineMultiDroneFormation/  Quadrotor9/Quadrotor/Translation/MATLAB Function1 ==
  data: q input; R output
function R = quat2rotm(q)
  R = eye(3);
  coder.extrinsic('quat2rotm.m');
  R = quat2rotm(q);
end

== matlab function ErskineMultiDroneFormation/  Quadrotor9/Quadrotor/calculate_wrench ==
  data: Omega_props input; thrust output; moments output; drone_params parameter; DroneID parameter
function [thrust, moments] =  invAllocation(Omega_props, drone_params, DroneID)

wrench = drone_params(DroneID).control.allocation_matrix*Omega_props.^2;

thrust = wrench(1);
moments = wrench(2:4);

== matlab function ErskineMultiDroneFormation/  Quadrotor9/add_noise ==
  settings: updateMethod=DISCRETE
  data: omega input; omega_n output size=3; q input; v input; p input; q_n output size=4; v_n output size=3; p_n output size=3; drone_params parameter; DroneID parameter
function [omega_n, q_n, v_n, p_n]= add_noise(omega,q,v,p, drone_params, DroneID)

omega_n = omega + drone_params(DroneID).sensor.gyroscope_noise*(rand(3,1)-0.5);

q_n = q + drone_params(DroneID).sensor.attitude_noise*(rand(4,1)-0.5);
q_n = q_n/norm(q_n);

v_n = v + drone_params(DroneID).sensor.velocity_noise*(rand(3,1)-0.5);

p_n = p + drone_params(DroneID).sensor.position_noise*(rand(3,1)-0.5);

end

== matlab function ErskineMultiDroneFormation/Formation Controller2/Camera ==
  settings: updateMethod=DISCRETE
  data: States input Bus: FormationStateBus; t input; bearings output; edges parameter; noisy_bearings output; depth output; noisy_depth output; camera_noise parameter; rng_seed parameter
function [bearings, noisy_bearings,depth, noisy_depth] = Cameras(States,t, edges, camera_noise, rng_seed)
%% Cameras(States, nDrones, edges)
% [bearings, noisy_bearings,depth, noisy_depth] = Cameras(States, nDrones, edges)

%% Setup Data Structures
drones = struct2cell(States);
bearings = zeros(3, length(edges));
noisy_bearings = zeros(3, length(edges));
depth = zeros(1, length(edges));
noisy_depth = zeros(1, length(edges));

rng(rng_seed + 1000*t);

%% Calculate Bearings
for i = 1:length(edges)
  out = edges(i,1);
  in = edges(i,2);
  
  %  drone_i = drones{out};
  %  drone_j = drones{in};
  
  Ri = quat2rotm(drones{out}.q');
  dp = drones{in}.p - drones{out}.p;
  depth(i) = norm(dp);
  bearings(:,i) = Ri' * dp/depth(i);
  
  % add noise
  perp1 = cross(bearings(:,i),rand(3,1));
  perp1 = perp1/norm(perp1);
  perp2 = cross(bearings(:,i),perp1);
  perp2 = perp2/norm(perp2);
  n1 = camera_noise.perp*2*(rand(1)-0.5)*perp1;
  n2 = camera_noise.perp*2*(rand(1)-0.5)*perp2;
  noisy_bearings(:,i) = bearings(:,i) + n1 + n2;
  noisy_bearings(:,i) = noisy_bearings(:,i)/norm(noisy_bearings(:,i));
  
  noisy_depth(i) = depth(i) + camera_noise.long_bias + ...
    2*camera_noise.long*(rand(1) - 0.5);
end

end

== matlab function ErskineMultiDroneFormation/  Quadrotor1/Quadrotor/calculate_wrench ==
  data: Omega_props input; thrust output; moments output; drone_params parameter; DroneID parameter
function [thrust, moments] =  invAllocation(Omega_props, drone_params, DroneID)

wrench = drone_params(DroneID).control.allocation_matrix*Omega_props.^2;

thrust = wrench(1);
moments = wrench(2:4);

== matlab function ErskineMultiDroneFormation/Formation Controller2/FormationControlFunction ==
  data: states input Bus: FormationStateBus; out output size=[4*nDrones]; B_desired input; B_forward input; B_measure input; d_measure input; init_guess input; nDrones parameter; result output; N_p parameter; dt_p parameter; edges parameter; control_type parameter
function [out, result] = FormationControlFunction(states, B_desired, B_forward, B_measure, d_measure, init_guess, nDrones, N_p, dt_p, edges, control_type)
%% ControlFunction
% the control u of a drone consists of [fz; omega]
% the output of this block is  out = [u1; u2; un]
% the result of a drone is [fz1; omega1; ...; fzn, omegan]
% the result of thisblock is [result1; ...; resultn]

% Determine if first iteration
if max(init_guess) < 0.001
  first_iter = true;
else
  first_iter = false;
end


% Function variables setup
out = zeros(nDrones*4,1);
result = init_guess;

coder.extrinsic('GradientBearingController');
coder.extrinsic('ForwardMPCFormationControl');
coder.extrinsic('CommunicatingMPCFormationControl');


%% Do Control
if control_type == 1 % Gradient Controller
  if first_iter
    disp(['Control type: Gradient'])
  end
  out = GradientBearingController(B_measure, B_desired, states, nDrones, edges);
  result = ones(nDrones*4*N_p, 1);
elseif control_type == 2 % Forward Desired MPC
  if first_iter
    for i = 1:4:length(init_guess)
      init_guess(i) = 10;
    end
    disp(['Control type: Forward MPC'])
  end
  [out, result] = ForwardMPCFormationControl(states, B_forward, B_measure, d_measure, init_guess, nDrones, N_p, dt_p, edges);
elseif control_type == 3 % Forward Desired MPC with Communication
  if first_iter
    for i = 1:4:length(init_guess)
      init_guess(i) = 10;
    end
    disp(['Control type: Forward MPC with Full Communication'])
  end
  [out, result] = CommunicatingMPCFormationControl(states, B_forward, B_measure, d_measure, init_guess, nDrones, N_p, dt_p, edges);
else
  error("Chosen Control Type is Invalid")
end


%% Processing of Results

return

== matlab function ErskineMultiDroneFormation/  Quadrotor10/Controller/Controller ==
  data: u input; p input size=3; v input size=3; q input size=4; omega input size=3; thrust output size=1; moments output size=3; control_type_param parameter; drone_params parameter; DroneID parameter; g parameter
function [thrust, moments] = controller(u, p, v, q, omega, control_type_param, drone_params, DroneID, g)

  thrust = 1; % set output dim
  moments = [0;0;0]; % set output dim
  
  coder.extrinsic('droneControl'); % link simulink to matlab function
  
  % do control
  [thrust, moments] = droneControl(u, p, v, q, omega, ...
    control_type_param, drone_params, DroneID, g);

end
